simulink model "dlbsTestHarnessGain"  (R2025b)
settings: Solver=FixedStepDiscrete  StartTime=0  StopTime=1  FixedStep=1  RelTol=1e-3
undefined symbols (not defined in the file or in its folder): dY, g, X
libraries: dlbsBlockGain x1, dlbsBlockExtractGradientGF x1, dlbsBlockInsertGradientGF x1
settings Model: Creator=lt6037  LastModifiedBy=lt6037

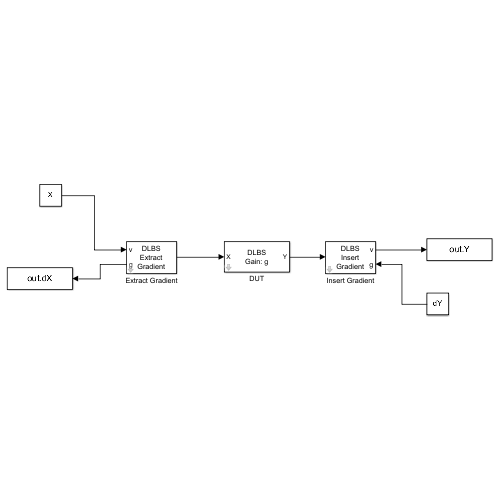
[thumbnail: Simulink's stored preview of the top-level diagram]
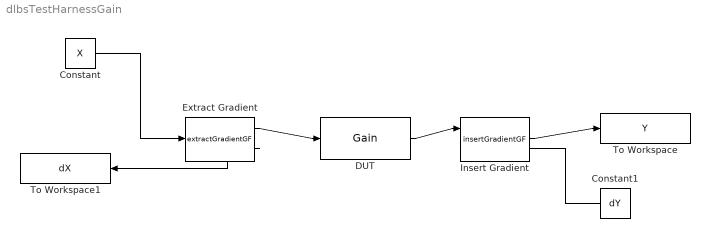
== system dlbsTestHarnessGain ==
  Constant : Constant  Value=X  VectorParams1D=off
  Constant1 : Constant  Value=dY  VectorParams1D=off
  DUT : dlbsBlockGain/Gain  Gain=g
  Extract Gradient : dlbsBlockExtractGradientGF/extractGradientGF
  Insert Gradient : dlbsBlockInsertGradientGF/insertGradientGF
  To Workspace : ToWorkspace  VariableName=Y  SaveFormat=Timeseries  SampleTime=-1
      settings: MaxDataPoints=1
  To Workspace1 : ToWorkspace  VariableName=dX  SaveFormat=Timeseries  SampleTime=-1
      settings: MaxDataPoints=1
  wires:
  Insert Gradient/1 -> To Workspace/1
  Extract Gradient/2 -> To Workspace1/1
  Constant1/1 -> Insert Gradient/2
  Constant/1 -> Extract Gradient/1
  Extract Gradient/1 -> DUT/1
  DUT/1 -> Insert Gradient/1
